simulink subsystem "ColdPlateSubsystem"  (R2025a)
settings: Solver=VariableStepAuto  StartTime=0.0  StopTime=10.0  RelTol=1e-3
undefined symbols (not defined in the file): TCoolantIn
libraries: fl_lib x5, nesl_utility x1
settings Model: Creator=epelster  LastModifiedBy=epelster

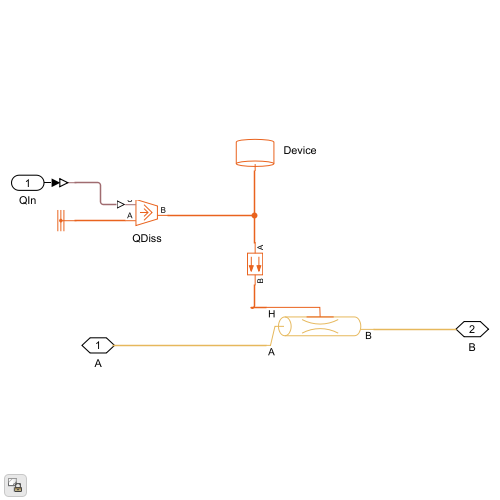
[thumbnail: Simulink's stored preview of the top-level diagram]
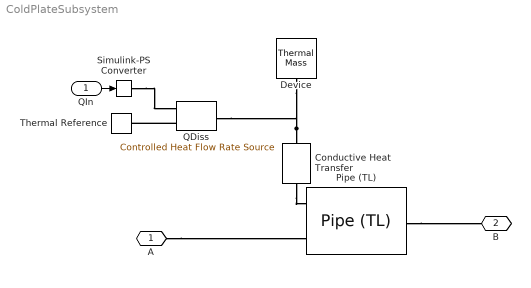
== system ColdPlateSubsystem ==
  QIn : Inport
  Conductive Heat Transfer : fl_lib/Thermal/Thermal Elements/Conductive Heat Transfer  thermal_type=foundation.enum.ConstantVariableTabulated.Constant  wall_geometry=foundation.enum.ConductionWallGeometry.Planar  area=cpDeviceSurfaceArea m^2  thickness=cpThickness mm  d_in=0.05 m  d_out=0.1 m  L=1 m  th_cond_min=10 W/(K*m)  th_cond=cpK W/(K*m)  th_cond_TLU=[413, 401, 392, 383, 371, 357, 342] W/(K*m)  temp_TLU=[200, 273, 400, 600, 800, 1000, 1200] K  T_specify=off  T_priority=None  T=0 K  T_nominal_specify=off  T_nominal_value=1  T_nominal_unit=K  Q_specify=off  Q_priority=None  Q=0 W  Q_nominal_specify=off  Q_nominal_value=1  Q_nominal_unit=W
  Device : fl_lib/Thermal/Thermal Elements/Thermal Mass  mass_type=foundation.enum.constant_variable.constant  mass=1 kg  sp_heat=447 J/(K*kg)  mass_min=1e-6 kg  num_ports=foundation.enum.numPorts2.one  m_specify=off  m_priority=High  m=1 kg  m_nominal_specify=off  m_nominal_value=1  m_nominal_unit=kg  T_specify=on  T_priority=High  T=TCoolantIn degC  T_nominal_specify=off  T_nominal_value=1  T_nominal_unit=K  Q_specify=off  Q_priority=None  Q=0 W  Q_nominal_specify=off  Q_nominal_value=1  Q_nominal_unit=W
  Pipe (TL) : fl_lib/Thermal Liquid/Elements/Pipe (TL)  length=channelLength m  area=channelArea mm^2  Dh=channelDh mm  length_add=0 m  roughness=channelRoughness m  Re_lam=2000  Re_tur=4000  shape_factor=64  Nu_lam=3.66  dynamic_compressibility=true  inertia=false  p0=pLoop bar  T0=TCoolantIn degC  mdot0=0 kg/s  p_nominal=0.101325 MPa  T_nominal=293.15 K
  QDiss : fl_lib/Thermal/Thermal Sources/Controlled Heat Flow Rate Source
  Simulink-PS Converter : nesl_utility/Simulink-PS Converter  PhysicalDomain=network_engine_domain  SubClassName=ps_input  LeftPortType=input  RightPortType=output  PseudoPeriodic=off  Frequencies=[]  NoiseDistribution=none  NoiseParameters=[]  Unit=W  AffineConversion=off  FilteringAndDerivatives=provide  SimscapeFilterOrder=1  InputFilterTimeConstant=0.001  UdotUserProvided=0
  Thermal Reference : fl_lib/Thermal/Thermal Elements/Thermal Reference
  A : PMIOPort  Side=Left
  B : PMIOPort  Port=2  Side=Right
  wires:
  QIn/1 -> Simulink-PS Converter/1
  connections:
  Conductive Heat Transfer/LConn1 -- Device/LConn1 -- QDiss/LConn1
  QDiss/RConn2 -- Thermal Reference/LConn1
  Conductive Heat Transfer/RConn1 -- Pipe (TL)/LConn2
  Pipe (TL)/RConn1 -- B/RConn1
  A/RConn1 -- Pipe (TL)/LConn1
  Simulink-PS Converter/RConn1 -- QDiss/RConn1
